simulink model "ssc_mass_spring_damper_sl_dbl"  (R2021b)
settings: Solver=VariableStepAuto  StartTime=0.0  StopTime=10.0  MaxStep=0.05  RelTol=1e-3  AbsTol=1e-3  EnableMultiTasking=on
PostLoadFcn:
  | m = 3.600;     % kg
  | k = 400;    % N/m
  | b = 10;      % Ns/m
libraries: fl_lib x11, nesl_utility x3
CloseFcn:
  | try,close(h1_ssc_mass_spring_damper_sl_dbl),end
  | clear h1_ssc_mass_spring_damper_sl_dbl
  | 
  | clear simlog_ssc_mass_spring_damper_sl_dbl
  | clear logsout_ssc_mass_spring_damper_sl_dbl
Description:
  | Double Mass-Spring-Damper in Simulink(R) and Simscape(TM)
settings Model: Creator=The MathWorks, Inc.  LastModifiedBy=The MathWorks, Inc.
settings SolverCC: AutoScaleAbsTol=off  AlgebraicLoopSolver=TrustRegion
settings DataIOCC: LimitDataPoints=on  SaveFormat=Array  ReturnWorkspaceOutputs=off  SignalLoggingName=logsout_ssc_mass_spring_damper_sl_dbl
settings OptimizationCC: LifeSpan=inf
settings DebuggingCC: SolverPrmCheckMsg=warning  AllowSymbolicDim=off  PregeneratedLibrarySubsystemCodeDiagnostic=none  SFUnexpectedBacktrackingDiag=warning  SFNoUnconditionalDefaultTransitionDiag=warning  SFExecutionAtInitializationDiag=none  SFMachineParentedDataDiag=warning  ArithmeticOperatorsInVariantConditions=warning
settings HardwareCC: ProdBitPerPointer=32  ProdBitPerSizeT=32  ProdBitPerPtrDiffT=32  ProdLargestAtomicFloat=None  ProdIntDivRoundTo=Undefined  ProdEndianess=Unspecified  ProdWordSize=32  ProdHWDeviceType=32-bit Generic
settings ModelReferenceCC: PropagateSignalLabelsOutOfModel=off
settings SFSimCC: SimUseLocalCustomCode=off  CustomCodeUndefinedFunction=UseInterfaceOnly
settings RTWCC: RTWUseLocalCustomCode=off
settings CodeAppCC: StateflowObjectComments=on
settings GRTTargetCC: TargetLangStandard=C89/C90 (ANSI)
settings ConfigComp: CovMetricSettings=dw  CovSaveCumulativeToWorkspaceVar=on  CovSaveSingleToWorkspaceVar=on  CovExternalEMLEnable=off  CovSFcnEnable=off
settings SimscapeCC: SimscapeLogType=all  SimscapeLogSimulationStatistics=on  SimscapeLogName=simlog_ssc_mass_spring_damper_sl_dbl  SimscapeLogDataHistory=10000

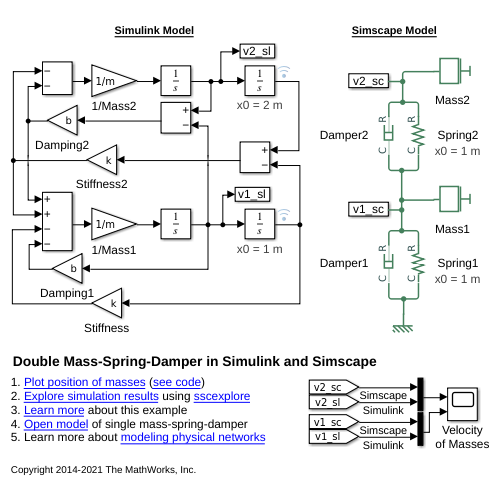
[thumbnail: Simulink's stored preview of the top-level diagram]
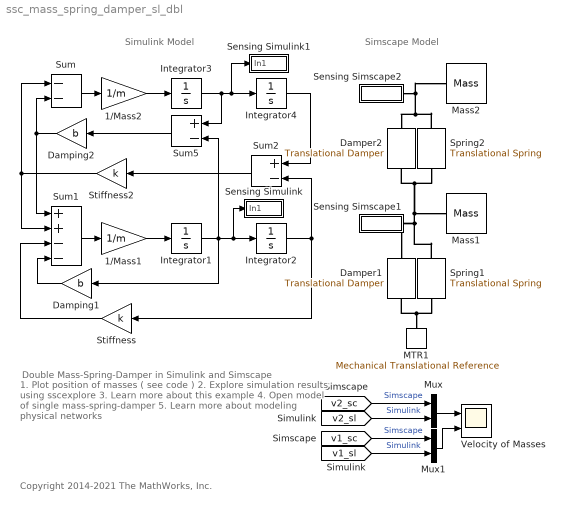
== system ssc_mass_spring_damper_sl_dbl ==
  note: 1. Plot position of masses ( see code )
      | 2. Explore simulation results using sscexplore
      | 3. Learn more about this example
      | 4. Open model of single mass-spring-damper
      | 5. Learn more about modeling physical networks
  note: Double Mass-Spring-Damper in Simulink and Simscape
  note: Simulink Model
  note: Simscape Model
  note: Copyright 2014-2021 The MathWorks, Inc.
  1/Mass1 : Gain  Gain=1/m  SaturateOnIntegerOverflow=on  OutDataTypeStr=Inherit: Same as input  ParamDataTypeStr=Inherit: Same as input
  1/Mass2 : Gain  Gain=1/m  SaturateOnIntegerOverflow=on  OutDataTypeStr=Inherit: Same as input  ParamDataTypeStr=Inherit: Same as input
  Damper1 : fl_lib/Mechanical/Translational Elements/Translational Damper  D=b N/(m/s)  v_specify=off  v_priority=High  v=0 m/s  v_nominal_specify=off  v_nominal_unit=m/s  v_nominal_value=1  f_specify=off  f_priority=High  f=0 N  f_nominal_specify=off  f_nominal_unit=N  f_nominal_value=1
  Damper2 : fl_lib/Mechanical/Translational Elements/Translational Damper  D=b N/(m/s)  v_specify=off  v_priority=High  v=0 m/s  v_nominal_specify=off  v_nominal_unit=m/s  v_nominal_value=1  f_specify=off  f_priority=High  f=0 N  f_nominal_specify=off  f_nominal_unit=N  f_nominal_value=1
  Damping1 : Gain  Gain=b  SaturateOnIntegerOverflow=on  OutDataTypeStr=Inherit: Same as input  ParamDataTypeStr=Inherit: Same as input
  Damping2 : Gain  Gain=b  SaturateOnIntegerOverflow=on  OutDataTypeStr=Inherit: Same as input  ParamDataTypeStr=Inherit: Same as input
  Integrator1 : Integrator
  Integrator2 : Integrator  InitialCondition=1
      settings: AttributesFormatString=x0 = %<InitialCondition> m
  Integrator3 : Integrator
  Integrator4 : Integrator  InitialCondition=2
      settings: AttributesFormatString=x0 = %<InitialCondition> m
  MTR1 : fl_lib/Mechanical/Translational Elements/Mechanical Translational Reference
  Mass1 : fl_lib/Mechanical/Translational Elements/Mass  mass=m kg  num_ports=foundation.enum.numPorts2.one  v_specify=off  v_priority=High  v=0 m/s  v_nominal_specify=off  v_nominal_unit=m/s  v_nominal_value=1  f_specify=off  f_priority=High  f=0 N  f_nominal_specify=off  f_nominal_unit=N  f_nominal_value=1
  Mass2 : fl_lib/Mechanical/Translational Elements/Mass  mass=m kg  num_ports=foundation.enum.numPorts2.one  v_specify=off  v_priority=High  v=0 m/s  v_nominal_specify=off  v_nominal_unit=m/s  v_nominal_value=1  f_specify=off  f_priority=High  f=0 N  f_nominal_specify=off  f_nominal_unit=N  f_nominal_value=1
  Mux : Mux  Inputs=2
  Mux1 : Mux  Inputs=2
  Sensing Simscape1 : Subsystem
      mask Display: disp('v1_sc')
  Sensing Simscape2 : Subsystem
      mask Display: disp('v2_sc')
  Sensing Simulink : Subsystem
      mask Display: disp('v1_sl')
  Sensing Simulink1 : Subsystem
      mask Display: disp('v2_sl')
  Spring1 : fl_lib/Mechanical/Translational Elements/Translational Spring  spr_rate=k N/m  v_specify=off  v_priority=High  v=0 m/s  v_nominal_specify=off  v_nominal_unit=m/s  v_nominal_value=1  f_specify=off  f_priority=High  f=0 N  f_nominal_specify=off  f_nominal_unit=N  f_nominal_value=1  x_specify=on  x_priority=High  x=1 m  x_nominal_specify=off  x_nominal_unit=m  x_nominal_value=1
      settings: AttributesFormatString=x0 = %<x> %<x_unit>
  Spring2 : fl_lib/Mechanical/Translational Elements/Translational Spring  spr_rate=k N/m  v_specify=off  v_priority=High  v=0 m/s  v_nominal_specify=off  v_nominal_unit=m/s  v_nominal_value=1  f_specify=off  f_priority=High  f=0 N  f_nominal_specify=off  f_nominal_unit=N  f_nominal_value=1  x_specify=on  x_priority=High  x=1 m  x_nominal_specify=off  x_nominal_unit=m  x_nominal_value=1
      settings: AttributesFormatString=x0 = %<x> %<x_unit>
  Stiffness : Gain  Gain=k  SaturateOnIntegerOverflow=on  OutDataTypeStr=Inherit: Same as input  ParamDataTypeStr=Inherit: Same as input
  Stiffness2 : Gain  Gain=k  SaturateOnIntegerOverflow=on  OutDataTypeStr=Inherit: Same as input  ParamDataTypeStr=Inherit: Same as input
  Sum : Sum  Inputs=--  InputSameDT=on  SaturateOnIntegerOverflow=on  OutDataTypeStr=Inherit: Same as first input
  Sum1 : Sum  Inputs=++--  InputSameDT=on  SaturateOnIntegerOverflow=on  OutDataTypeStr=Inherit: Same as first input
  Sum2 : Sum  Inputs=+-  InputSameDT=on  SaturateOnIntegerOverflow=on  OutDataTypeStr=Inherit: Same as first input
  Sum5 : Sum  Inputs=+-  InputSameDT=on  SaturateOnIntegerOverflow=on  OutDataTypeStr=Inherit: Same as first input
  Velocity of Masses : Scope  NumInputPorts=2
  wires:
  1/Mass1/1 -> Integrator1/1
  Sum1/1 -> 1/Mass1/1
  Sum5/1 -> Damping2/1
  Damping2/1 -> Sum/2, Sum1/1
  1/Mass2/1 -> Integrator3/1
  Sum/1 -> 1/Mass2/1
  Integrator4/1 -> Sum2/1
  Integrator3/1 -> Sensing Simulink1/1(In1), Integrator4/1, Sum5/1
  Sum2/1 -> Stiffness2/1
  Stiffness2/1 -> Sum1/2, Sum/1
  Damping1/1 -> Sum1/4
  Stiffness/1 -> Sum1/3
  Integrator2/1 -> Sum2/2, Stiffness/1
  Integrator1/1 -> Sum5/2, Sensing Simulink/1(In1), Integrator2/1, Damping1/1
  Mux/1 -> Velocity of Masses/1
  [v2_sc] -> Mux/1  "Simscape"
  [v2_sl] -> Mux/2  "Simulink"
  Mux1/1 -> Velocity of Masses/2
  [v1_sc] -> Mux1/1  "Simscape"
  [v1_sl] -> Mux1/2  "Simulink"
  connections:
  Spring1/RConn1 -- Damper1/RConn1 -- MTR1/LConn1
  Spring2/RConn1 -- Sensing Simscape1/LConn1 -- Spring1/LConn1 -- Damper1/LConn1 -- Mass1/LConn1 -- Damper2/RConn1
  Spring2/LConn1 -- Sensing Simscape2/LConn1 -- Mass2/LConn1 -- Damper2/LConn1

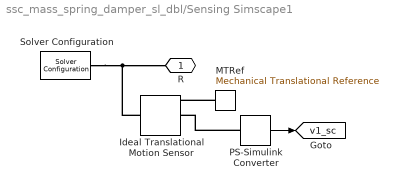
== system ssc_mass_spring_damper_sl_dbl/Sensing Simscape1 ==
  Ideal Translational Motion Sensor : fl_lib/Mechanical/Mechanical Sensors/Ideal Translational Motion Sensor  offset=1 m
  MTRef : fl_lib/Mechanical/Translational Elements/Mechanical Translational Reference
  PS-Simulink Converter : nesl_utility/PS-Simulink Converter  PhysicalDomain=network_engine_domain  SubClassName=ps_output  LeftPortType=input  RightPortType=output  PseudoPeriodic=off  Frequencies=[]  Unit=1  AffineConversion=off
      settings: SourceProductBaseCode=PW,SS
  Solver Configuration : nesl_utility/Solver Configuration  PhysicalDomain=network_engine_domain  SubClassName=solver  LeftPortType=input  RightPortType=generic  Tones=[]  Harmonics=[]  SimulateNoise=off  Profile=off  UseLocalSampling=off  EnableSwitchedLinearOptims=on  FrequencyDomain=off  UseCCode=off  RelTol=0.001  AbsTol=1e-06  MinStep=1e-09  ToWorkspace=off  RevertToSquareIcSolve=off  NumHomotopyIterations=100  PhasorMode=off  PhasorModeNumHarmonics=1  DoDC=off  ResidualTolerance=1e-9  UseLocalSolver=off  LocalSolverChoice=NE_BACKWARD_EULER_ADVANCER  LocalSolverSampleTime=.001  DoFixedCost=off  MaxNonlinIter=12  MaxModeIter=2  ComputeImpulses=off  ImpulseIterations=2  LinearAlgebra=auto  EquationFormulation=NE_TIME_EF  DelaysMemoryBudget=1024  AutomaticFiltering=on  FilteringTimeConstant=0.001  PartitionStorageMethod=AS_NEEDED  PartitionMemoryBudget=1024  PartitionMethod=FAST
      settings: SourceProductBaseCode=PW,SS
  R : PMIOPort  Side=Left
  tag scope: v1_sc=global
  wires:
  PS-Simulink Converter/1 -> [v1_sc]
  connections:
  MTRef/LConn1 -- Ideal Translational Motion Sensor/RConn1
  PS-Simulink Converter/LConn1 -- Ideal Translational Motion Sensor/RConn2
  Ideal Translational Motion Sensor/LConn1 -- Solver Configuration/RConn1 -- R/RConn1

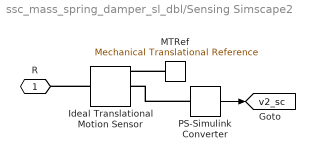
== system ssc_mass_spring_damper_sl_dbl/Sensing Simscape2 ==
  Ideal Translational Motion Sensor : fl_lib/Mechanical/Mechanical Sensors/Ideal Translational Motion Sensor  offset=1 m
  MTRef : fl_lib/Mechanical/Translational Elements/Mechanical Translational Reference
  PS-Simulink Converter : nesl_utility/PS-Simulink Converter  PhysicalDomain=network_engine_domain  SubClassName=ps_output  LeftPortType=input  RightPortType=output  PseudoPeriodic=off  Frequencies=[]  Unit=1  AffineConversion=off
      settings: SourceProductBaseCode=PW,SS
  R : PMIOPort  Side=Left
  tag scope: v2_sc=global
  wires:
  PS-Simulink Converter/1 -> [v2_sc]
  connections:
  Ideal Translational Motion Sensor/LConn1 -- R/RConn1
  PS-Simulink Converter/LConn1 -- Ideal Translational Motion Sensor/RConn2
  MTRef/LConn1 -- Ideal Translational Motion Sensor/RConn1

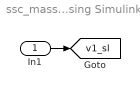
== system ssc_mass_spring_damper_sl_dbl/Sensing Simulink ==
  In1 : Inport
  tag scope: v1_sl=global
  wires:
  In1/1 -> [v1_sl]

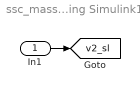
== system ssc_mass_spring_damper_sl_dbl/Sensing Simulink1 ==
  In1 : Inport
  tag scope: v2_sl=global
  wires:
  In1/1 -> [v2_sl]
